simulink model "body_dynamics"  (Simulink 7.1)
settings: Solver=ode45  StartTime=0.0  StopTime=10.0  RelTol=1e-3
undefined symbols (not defined in the file or in its folder): Iinv
libraries: simulink x12
settings Model: Creator=cb09214  LastModifiedBy=ranjan
settings DebuggingCC: SaveWithParameterizedLinksMsg=none
settings GRTTargetCC: TargetFcnLib=ansi_tfl_tmw.mat

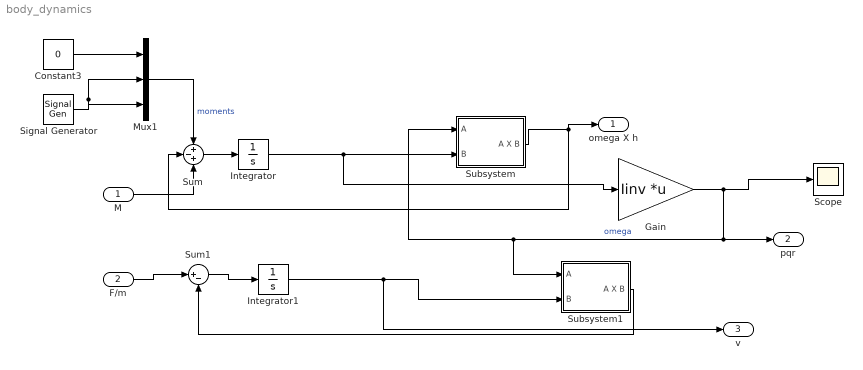
== system body_dynamics ==
  M : Inport  OutDataType=sfix(16)  OutScaling=2^0
  F/m : Inport  Port=2  OutDataType=sfix(16)  OutScaling=2^0
  Constant3 : Constant  Value=0  OutDataType=sfix(16)  OutScaling=2^0
  Gain : Gain  Gain=Iinv  Multiplication=Matrix(K*u)  ParameterDataType=sfix(16)  ParameterScaling=2^0  OutDataType=sfix(16)  OutScaling=2^0
  Integrator : Integrator
  Integrator1 : Integrator
  Mux1 : Mux  Inputs=3
  Scope : Scope
  Signal Generator : SignalGenerator
  Subsystem : Subsystem
  Subsystem1 : Subsystem
  Sum : Sum  Inputs=+-+  OutDataType=sfix(16)  OutScaling=2^0
  Sum1 : Sum  Inputs=|+-  OutDataType=sfix(16)  OutScaling=2^0
  omega X h : Outport  OutDataType=sfix(16)  OutScaling=2^0
  pqr : Outport  Port=2  OutDataType=sfix(16)  OutScaling=2^0
  v : Outport  Port=3  OutDataType=sfix(16)  OutScaling=2^0
  wires:
  Subsystem/1(A X B) -> omega X h/1, Sum/2
  Integrator/1 -> Subsystem/2(B), Gain/1
  Sum/1 -> Integrator/1
  M/1 -> Sum/3
  Signal Generator/1 -> Mux1/2, Mux1/3
  Constant3/1 -> Mux1/1
  Mux1/1 -> Sum/1  "moments"
  Gain/1 -> Scope/1, pqr/1, Subsystem/1(A), Subsystem1/1(A)  "omega"
  Subsystem1/1(A X B) -> Sum1/2
  F/m/1 -> Sum1/1
  Sum1/1 -> Integrator1/1
  Integrator1/1 -> Subsystem1/2(B), v/1

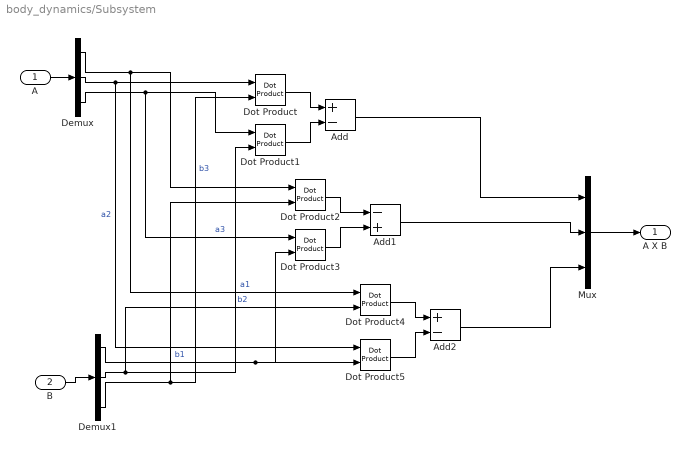
== system body_dynamics/Subsystem ==
  A : Inport  OutDataType=sfix(16)  OutScaling=2^0
  B : Inport  Port=2  OutDataType=sfix(16)  OutScaling=2^0
  Add : Sum  Inputs=+-  OutDataType=sfix(16)  OutScaling=2^-10
  Add1 : Sum  Inputs=-+  OutDataType=sfix(16)  OutScaling=2^-10
  Add2 : Sum  Inputs=+-  OutDataType=sfix(16)  OutScaling=2^-10
  Demux : Demux  Outputs=3
  Demux1 : Demux  Outputs=3
  Dot Product{,1..5} (6 alike) : simulink/Math Operations/Dot Product  InputSameDT=on  OutDataType=sfix(16)  OutScaling=2^-10  DoSatur=off
  Mux : Mux  Inputs=3
  A X B : Outport  OutDataType=sfix(16)  OutScaling=2^0
  wires:
  Demux/2 -> Dot Product/1, Dot Product5/1  "a2"
  Demux1/3 -> Dot Product/2, Dot Product2/2  "b3"
  Demux/3 -> Dot Product1/1, Dot Product3/1  "a3"
  Demux1/2 -> Dot Product1/2, Dot Product4/2  "b2"
  Dot Product/1 -> Add/1
  Dot Product1/1 -> Add/2
  Add/1 -> Mux/1
  Demux/1 -> Dot Product2/1, Dot Product4/1  "a1"
  Demux1/1 -> Dot Product3/2, Dot Product5/2  "b1"
  Dot Product2/1 -> Add1/1
  Dot Product3/1 -> Add1/2
  Add1/1 -> Mux/2
  Dot Product4/1 -> Add2/1
  Dot Product5/1 -> Add2/2
  Add2/1 -> Mux/3
  A/1 -> Demux/1
  B/1 -> Demux1/1
  Mux/1 -> A X B/1

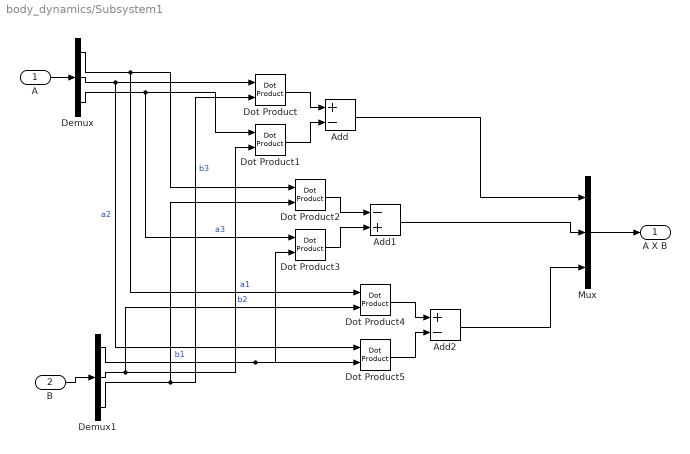
== system body_dynamics/Subsystem1 ==
  A : Inport  OutDataType=sfix(16)  OutScaling=2^0
  B : Inport  Port=2  OutDataType=sfix(16)  OutScaling=2^0
  Add : Sum  Inputs=+-  OutDataType=sfix(16)  OutScaling=2^-10
  Add1 : Sum  Inputs=-+  OutDataType=sfix(16)  OutScaling=2^-10
  Add2 : Sum  Inputs=+-  OutDataType=sfix(16)  OutScaling=2^-10
  Demux : Demux  Outputs=3
  Demux1 : Demux  Outputs=3
  Dot Product{,1..5} (6 alike) : simulink/Math Operations/Dot Product  InputSameDT=on  OutDataType=sfix(16)  OutScaling=2^-10  DoSatur=off
  Mux : Mux  Inputs=3
  A X B : Outport  OutDataType=sfix(16)  OutScaling=2^0
  wires:
  Demux/2 -> Dot Product/1, Dot Product5/1  "a2"
  Demux1/3 -> Dot Product/2, Dot Product2/2  "b3"
  Demux/3 -> Dot Product1/1, Dot Product3/1  "a3"
  Demux1/2 -> Dot Product1/2, Dot Product4/2  "b2"
  Dot Product/1 -> Add/1
  Dot Product1/1 -> Add/2
  Add/1 -> Mux/1
  Demux/1 -> Dot Product2/1, Dot Product4/1  "a1"
  Demux1/1 -> Dot Product3/2, Dot Product5/2  "b1"
  Dot Product2/1 -> Add1/1
  Dot Product3/1 -> Add1/2
  Add1/1 -> Mux/2
  Dot Product4/1 -> Add2/1
  Dot Product5/1 -> Add2/2
  Add2/1 -> Mux/3
  A/1 -> Demux/1
  B/1 -> Demux1/1
  Mux/1 -> A X B/1
